simulink model "simulacion"  (R2022b)
settings: Solver=VariableStepAuto  StartTime=0.0  StopTime=10  RelTol=1e-3
values from neighbouring files (symbols this model uses):
  beta = gamma*2*I    (= 0.0001265)    [parametros.m]
  db = 4.2/100    (= 0.042)    [parametros.m]
  dc = 5/100    (= 0.05)    [parametros.m]
  dm = 13.1/100    (= 0.131)    [parametros.m]
  g = 9.81    [parametros.m]
  I = 1.1e-4    (= 0.00011)    [parametros.m]
  K = 0.001    [parametros.m]
  mb = 7.38/1000    (= 0.00738)    [parametros.m]
  mc = 2.07/1000    (= 0.00207)    [parametros.m]
  mm = (3.2+1.28)/1000    (= 0.00448)    [parametros.m]
undefined symbols (not defined in the file or in its folder): polo_vhs_abs
libraries: slpidlib x2
settings Model: Creator=TAURET  LastModifiedBy=danie
settings DataIOCC: Refine=100
settings ModelReferenceCC: EnableRefExpFcnMdlSchedulingChecks=on

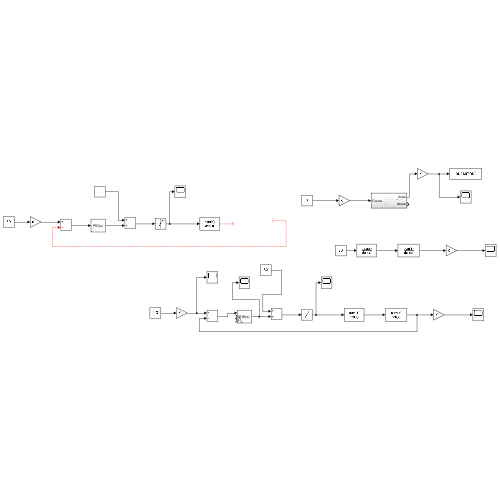
[thumbnail: Simulink's stored preview of the top-level diagram]
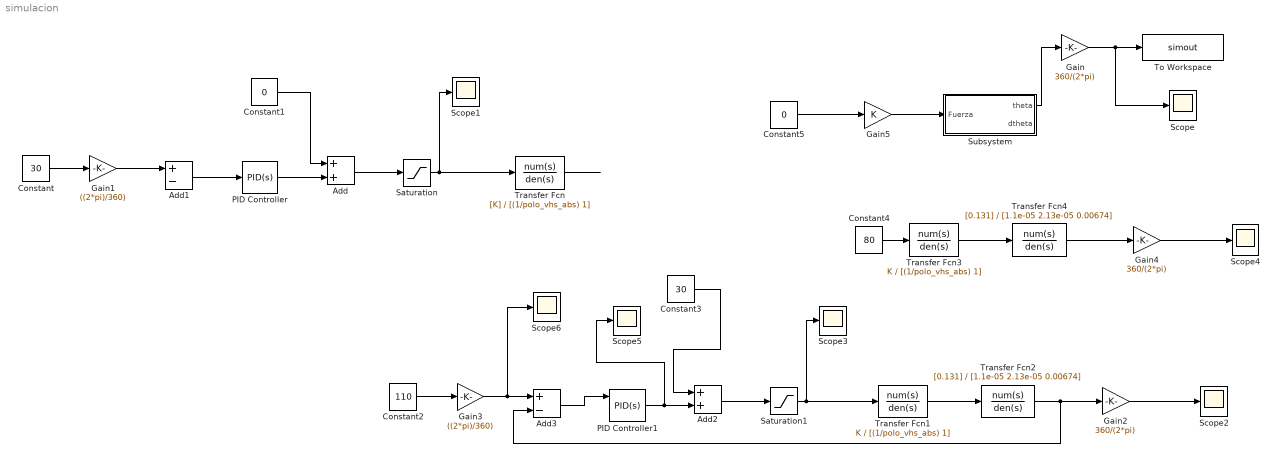
== system simulacion ==
  Add : Sum
  Add1 : Sum  Inputs=+-
  Add2 : Sum
  Add3 : Sum  Inputs=+-
  Constant : Constant  Value=30
  Constant1 : Constant  Value=0
  Constant2 : Constant  Value=110
  Constant3 : Constant  Value=30
  Constant4 : Constant  Value=80
  Constant5 : Constant  Value=0
  Gain : Gain  Gain=360/(2*pi)
  Gain1 : Gain  Gain=((2*pi)/360)
  Gain2 : Gain  Gain=360/(2*pi)
  Gain3 : Gain  Gain=((2*pi)/360)
  Gain4 : Gain  Gain=360/(2*pi)
  Gain5 : Gain  Gain=K
  PID Controller : slpidlib/PID Controller  Controller=PID  Form=Parallel  TimeDomain=Continuous-time  UseExternalTs=off  SampleTime=-1  IntegratorMethod=Forward Euler  FilterMethod=Forward Euler  ControllerParametersSource=internal  P=1  I=1  UseKiTs=off  D=0  N=0  UseFilter=on  TunerSelectOption=Transfer Function Based (PID Tuner App)  InitialConditionSource=internal  InitialConditionForIntegrator=0  InitialConditionForFilter=0  DifferentiatorICPrevScaledInput=0  ExternalReset=none  TrackingMode=off  Kt=1  LimitOutput=off  SatLimitsSource=internal  UpperSaturationLimit=inf  LowerSaturationLimit=-inf  LinearizeAsGain=on  AntiWindupMode=none  Kb=1  LimitIntegrator=off  UpperIntegratorSaturationLimit=inf  LowerIntegratorSaturationLimit=-inf  POutMin=[]  POutMax=[]  IOutMin=[]  IOutMax=[]  DOutMin=[]  DOutMax=[]  NOutMin=[]  NOutMax=[]  SumOutMin=[]  SumOutMax=[]  SaturationOutMin=[]  SaturationOutMax=[]  PParamMin=[]  PParamMax=[]  IParamMin=[]  IParamMax=[]  DParamMin=[]  DParamMax=[]  NParamMin=[]  NParamMax=[]  KbParamMin=[]  KbParamMax=[]  KtParamMin=[]  KtParamMax=[]  KbOutMin=[]  KbOutMax=[]  KtOutMin=[]  KtOutMax=[]  IntegratorOutMin=[]  IntegratorOutMax=[]  FilterOutMin=[]  FilterOutMax=[]  SumI1OutMin=[]  SumI1OutMax=[]  SumI2OutMin=[]  SumI2OutMax=[]  SumI3OutMin=[]  SumI3OutMax=[]  SumI4OutMin=[]  SumI4OutMax=[]  SumDOutMin=[]  SumDOutMax=[]  DifferentiatorOutMin=[]  DifferentiatorOutMax=[]  FilterDiffOutCoefMin=[]  FilterDiffOutCoefMax=[]  ReciprocalOutMin=[]  ReciprocalOutMax=[]  SumDenOutMin=[]  SumDenOutMax=[]  SumNumOutMin=[]  SumNumOutMax=[]  DivideOutMin=[]  DivideOutMax=[]  UdiffTsProdOutMin=[]  UdiffTsProdOutMax=[]  NTsProdOutMin=[]  NTsProdOutMax=[]  UintegralTsProdOutMin=[]  UintegralTsProdOutMax=[]  UngainTsProdOutMin=[]  UngainTsProdOutMax=[]  ClampingZeroOutDataTypeStr=Inherit: Inherit via back propagation  ClampingZeroOutMin=[]  ClampingZeroOutMax=[]  FilterDenConstantOutDataTypeStr=Inherit: Inherit via back propagation  FilterDenConstantOutMin=[]  FilterDenConstantOutMax=[]  PCopyOutDataTypeStr=Inherit: Inherit via back propagation  PCopyOutMin=[]  PCopyOutMax=[]  NCopyOutDataTypeStr=Inherit: Inherit via back propagation  NCopyOutMin=[]  NCopyOutMax=[]  IntegratorContinuousStateAttributes=''  IntegratorStateMustResolveToSignalObject=off  IntegratorRTWStateStorageClass=Auto  FilterContinuousStateAttributes=''  FilterStateMustResolveToSignalObject=off  FilterRTWStateStorageClass=Auto  ParallelPVariant=InternalParameters  IdealPVariant=Disabled  IVariant=InternalParameters  DVariant=InternalParameters  IntegratorVariant=Continuous  SatVariant=Disabled  AWVariant=Passthrough  PCopyVariant=Disabled  TRVariant=Disabled  FdbkBlocksVariant=Forward  IdealPFdbkVariant=Disabled  SatFdbkVariant=Disabled  DerivativeFilterVariant=ContFilter  NVariant=InternalParameters  NCopyVariant=Disabled  FilterICVariant=InternalICsFilter  IntegratorICVariant=InternalICs  ExternalResetVariant=Disabled  TRSumVariant=Passthrough  SumFdbkVariant=Disabled  SumVariant=Sum_PID  TsampFilterVariant=InternalTs  TsampNgainVariant=Passthrough  TsampIntegralVariant=Passthrough  ExternalSaturationOutDataTypeStr=Inherit: Same as second input
  PID Controller1 : slpidlib/PID Controller  Controller=PID  Form=Parallel  TimeDomain=Continuous-time  UseExternalTs=off  SampleTime=-1  IntegratorMethod=Forward Euler  FilterMethod=Forward Euler  ControllerParametersSource=internal  P=25.1032763477177  I=229.841028329094  UseKiTs=on  D=-5.16676671736803  N=4.24370556440195  UseFilter=on  TunerSelectOption=Transfer Function Based (PID Tuner App)  InitialConditionSource=external  InitialConditionForIntegrator=0  InitialConditionForFilter=0  DifferentiatorICPrevScaledInput=0  ExternalReset=none  TrackingMode=off  Kt=1  LimitOutput=off  SatLimitsSource=internal  UpperSaturationLimit=inf  LowerSaturationLimit=-inf  LinearizeAsGain=on  AntiWindupMode=none  Kb=1  LimitIntegrator=off  UpperIntegratorSaturationLimit=inf  LowerIntegratorSaturationLimit=-inf  POutMin=[]  POutMax=[]  IOutMin=[]  IOutMax=[]  DOutMin=[]  DOutMax=[]  NOutMin=[]  NOutMax=[]  SumOutMin=[]  SumOutMax=[]  SaturationOutMin=[]  SaturationOutMax=[]  PParamMin=[]  PParamMax=[]  IParamMin=[]  IParamMax=[]  DParamMin=[]  DParamMax=[]  NParamMin=[]  NParamMax=[]  KbParamMin=[]  KbParamMax=[]  KtParamMin=[]  KtParamMax=[]  KbOutMin=[]  KbOutMax=[]  KtOutMin=[]  KtOutMax=[]  IntegratorOutMin=[]  IntegratorOutMax=[]  FilterOutMin=[]  FilterOutMax=[]  SumI1OutMin=[]  SumI1OutMax=[]  SumI2OutMin=[]  SumI2OutMax=[]  SumI3OutMin=[]  SumI3OutMax=[]  SumI4OutMin=[]  SumI4OutMax=[]  SumDOutMin=[]  SumDOutMax=[]  DifferentiatorOutMin=[]  DifferentiatorOutMax=[]  FilterDiffOutCoefMin=[]  FilterDiffOutCoefMax=[]  ReciprocalOutMin=[]  ReciprocalOutMax=[]  SumDenOutMin=[]  SumDenOutMax=[]  SumNumOutMin=[]  SumNumOutMax=[]  DivideOutMin=[]  DivideOutMax=[]  UdiffTsProdOutMin=[]  UdiffTsProdOutMax=[]  NTsProdOutMin=[]  NTsProdOutMax=[]  UintegralTsProdOutMin=[]  UintegralTsProdOutMax=[]  UngainTsProdOutMin=[]  UngainTsProdOutMax=[]  ClampingZeroOutDataTypeStr=Inherit: Inherit via back propagation  ClampingZeroOutMin=[]  ClampingZeroOutMax=[]  FilterDenConstantOutDataTypeStr=Inherit: Inherit via back propagation  FilterDenConstantOutMin=[]  FilterDenConstantOutMax=[]  PCopyOutDataTypeStr=Inherit: Inherit via back propagation  PCopyOutMin=[]  PCopyOutMax=[]  NCopyOutDataTypeStr=Inherit: Inherit via back propagation  NCopyOutMin=[]  NCopyOutMax=[]  IntegratorContinuousStateAttributes=''  IntegratorStateMustResolveToSignalObject=off  IntegratorRTWStateStorageClass=Auto  FilterContinuousStateAttributes=''  FilterStateMustResolveToSignalObject=off  FilterRTWStateStorageClass=Auto  ParallelPVariant=InternalParameters  IdealPVariant=Disabled  IVariant=InternalParameters  DVariant=InternalParameters  IntegratorVariant=Continuous  SatVariant=Disabled  AWVariant=Passthrough  PCopyVariant=Disabled  TRVariant=Disabled  FdbkBlocksVariant=Forward  IdealPFdbkVariant=Disabled  SatFdbkVariant=Disabled  DerivativeFilterVariant=ContFilter  NVariant=InternalParameters  NCopyVariant=Disabled  FilterICVariant=ExternalICs  IntegratorICVariant=ExternalICs  ExternalResetVariant=Disabled  TRSumVariant=Passthrough  SumFdbkVariant=Disabled  SumVariant=Sum_PID  TsampFilterVariant=InternalTs  TsampNgainVariant=Passthrough  TsampIntegralVariant=Passthrough  ExternalSaturationOutDataTypeStr=Inherit: Same as second input
  Saturation : Saturate  UpperLimit=59  LowerLimit=0
  Saturation1 : Saturate  UpperLimit=59  LowerLimit=0
  Scope{,1..6} (7 alike) : Scope
  Subsystem : Subsystem
  To Workspace : ToWorkspace  VariableName=simout  SaveFormat=Timeseries  SampleTime=-1
  Transfer Fcn : TransferFcn  Numerator=[K]  Denominator=[(1/polo_vhs_abs) 1]
  Transfer Fcn1 : TransferFcn  Numerator=K  Denominator=[(1/polo_vhs_abs) 1]
  Transfer Fcn2 : TransferFcn  Numerator=[0.131]  Denominator=[1.1e-05 2.13e-05 0.00674]
  Transfer Fcn3 : TransferFcn  Numerator=K  Denominator=[(1/polo_vhs_abs) 1]
  Transfer Fcn4 : TransferFcn  Numerator=[0.131]  Denominator=[1.1e-05 2.13e-05 0.00674]
  wires:
  Subsystem/1(theta) -> Gain/1
  Gain/1 -> To Workspace/1, Scope/1
  Transfer Fcn1/1 -> Transfer Fcn2/1
  Constant2/1 -> Gain3/1
  Add3/1 -> PID Controller1/1
  Gain3/1 -> Scope6/1, Add3/1
  Constant3/1 -> Add2/1
  Add2/1 -> Saturation1/1
  PID Controller1/1 -> Scope5/1, Add2/2
  Saturation1/1 -> Transfer Fcn1/1, Scope3/1
  Transfer Fcn2/1 -> Add3/2, Gain2/1
  Gain2/1 -> Scope2/1
  Transfer Fcn3/1 -> Transfer Fcn4/1
  Transfer Fcn4/1 -> Gain4/1
  Gain4/1 -> Scope4/1
  Constant4/1 -> Transfer Fcn3/1
  ? -> Add1/2
  PID Controller/1 -> Add/2
  Add/1 -> Saturation/1
  Constant1/1 -> Add/1
  Add1/1 -> PID Controller/1
  Constant/1 -> Gain1/1
  Transfer Fcn/1 -> ?
  Gain1/1 -> Add1/1
  Saturation/1 -> Transfer Fcn/1, Scope1/1
  Constant5/1 -> Gain5/1
  Gain5/1 -> Subsystem/1(Fuerza)

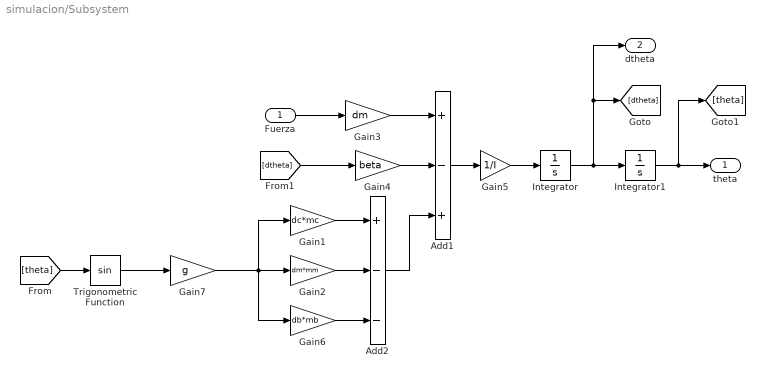
== system simulacion/Subsystem ==
  Fuerza : Inport
  Add1 : Sum  Inputs=+-+
  Add2 : Sum  Inputs=+--
  Gain1 : Gain  Gain=dc*mc
  Gain2 : Gain  Gain=dm*mm
  Gain3 : Gain  Gain=dm
  Gain4 : Gain  Gain=beta
  Gain5 : Gain  Gain=1/I
  Gain6 : Gain  Gain=db*mb
  Gain7 : Gain  Gain=g
  Integrator : Integrator
  Integrator1 : Integrator  InitialCondition=1.57
  Trigonometric Function : Trigonometry
  theta : Outport
  dtheta : Outport  Port=2
  wires:
  Gain4/1 -> Add1/2
  Gain5/1 -> Integrator/1
  Add1/1 -> Gain5/1
  [dtheta] -> Gain4/1
  [theta] -> Trigonometric Function/1
  Integrator/1 -> dtheta/1, [dtheta], Integrator1/1
  Integrator1/1 -> [theta], theta/1
  Fuerza/1 -> Gain3/1
  Gain1/1 -> Add2/1
  Gain2/1 -> Add2/2
  Gain6/1 -> Add2/3
  Add2/1 -> Add1/3
  Trigonometric Function/1 -> Gain7/1
  Gain3/1 -> Add1/1
  Gain7/1 -> Gain6/1, Gain2/1, Gain1/1
